simulink model "TRMS_MRAC_Node"  (R2024a)
settings: Solver=ode1  StartTime=0.0  StopTime=inf  FixedStep=0.01  RelTol=1e-3
model workspace (MAT data in the model file):
  alpha_gain = Simulink.Parameter
  alpha_gain.Value = 0.98
  alpha_gain.Complexity = 'real'
  alpha_gain.Dimensions = [1 1]
  alpha_gain.DataType = 'auto'
undefined symbols (not defined in the file or in its folder): A, B, C, D, DiscIntNeverNeededParam, P, pin_number, state, theta_theta
libraries: ros2lib x17, dspstat3 x1, sharedutil x1
settings Model: Creator=dsai9  LastModifiedBy=dsai9
settings OptimizationCC: EnhancedBackFolding=on  PassReuseOutputArgsAs=Individual arguments  ZeroExternalMemoryAtStartup=off  ZeroInternalMemoryAtStartup=off  MaxStackSize=64  OptimizeBlockOrder=speed  DifferentSizesBufferReuse=on  OptimizationCustomize=off  EfficientTunableParamExpr=on
settings DebuggingCC: ParameterTunabilityLossMsg=error
settings SFSimCC: MATLABDynamicMemAlloc=off
settings RTWCC: Description=Embedded Coder  SystemTargetFile=ert.tlc  HardwareBoard=Robot Operating System 2 (ROS 2)  TLCOptions="-aInlineSetEventsForThisBaseRateFcn=TLC_FALSE -aSuppressMultiTaskScheduler=TLC_FALSE  -aRateBasedStepFcn=0"  TemplateMakefile=ert_default_tmf  Toolchain=Colcon Tools  TargetLang=C++
settings CodeAppCC: ForceParamTrailComments=on  IgnoreCustomStorageClasses=off  OperatorAnnotations=on  SimulinkDataObjDesc=on  SFDataObjDesc=on  InsertBlockDesc=on
settings ERTTargetCC: CodeInterfacePackaging=C++ class  SupportContinuousTime=on  RootIOFormat=Structure reference

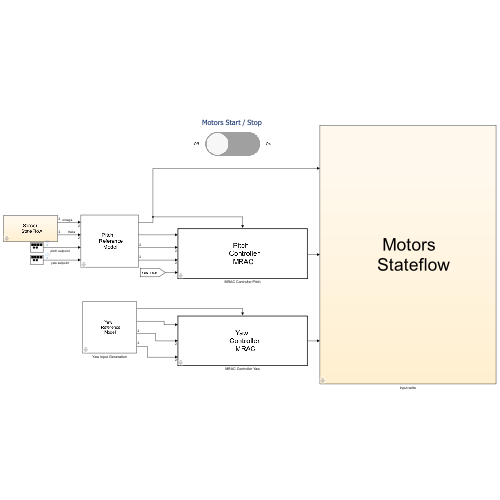
[thumbnail: Simulink's stored preview of the top-level diagram]
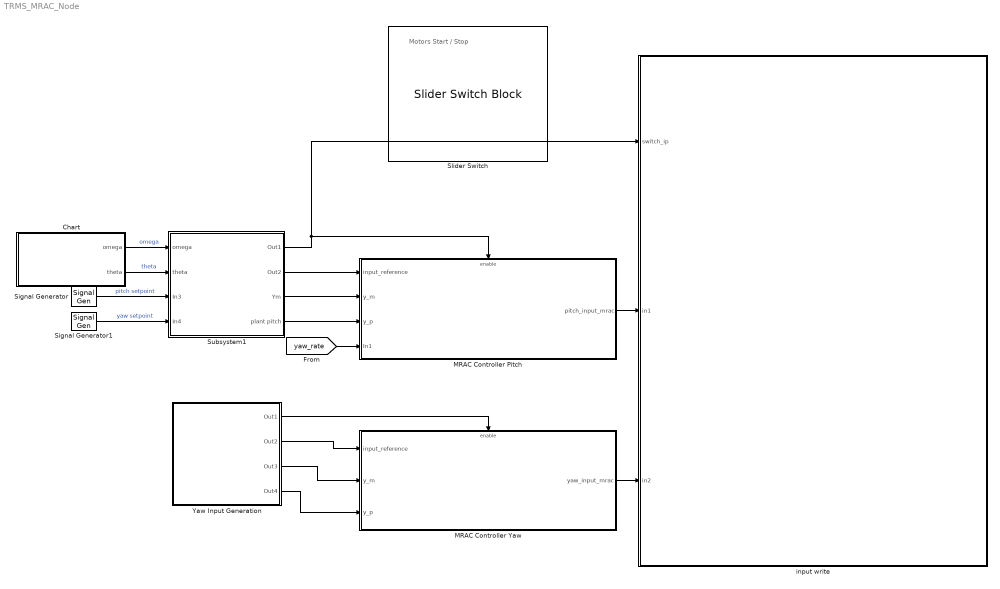
== system TRMS_MRAC_Node ==
  note: Motors Start / Stop
  Chart : Stateflow chart  TreatAsAtomicUnit=on
  MRAC Controller Pitch : Subsystem
  MRAC Controller Yaw : Subsystem
  Signal Generator : SignalGenerator  Amplitude=0  Frequency=0.5  Units=rad/sec
  Signal Generator1 : SignalGenerator  Amplitude=0  Frequency=0.5  Units=rad/sec
  Slider Switch : SliderSwitchBlock  LabelPosition=Hide
      settings: Values={{'Off', 'On'}, [0 1]}
  Subsystem1 : Subsystem
  Yaw Input Generation : Subsystem
  input write : Stateflow chart  TreatAsAtomicUnit=on
  wires:
  Yaw Input Generation/1(Out1) -> MRAC Controller Yaw/Enable
  Yaw Input Generation/2(Out2) -> MRAC Controller Yaw/1(input_reference)
  Yaw Input Generation/3(Out3) -> MRAC Controller Yaw/2(y_m)
  Yaw Input Generation/4(Out4) -> MRAC Controller Yaw/3(y_p)
  MRAC Controller Pitch/1(pitch_input_mrac) -> input write/2(in1)
  MRAC Controller Yaw/1(yaw_input_mrac) -> input write/3(in2)
  Chart/1(omega) -> Subsystem1/1(omega)  "omega"
  Chart/2(theta) -> Subsystem1/2(theta)  "theta"
  Signal Generator/1 -> Subsystem1/3(In3)  "pitch setpoint"
  Signal Generator1/1 -> Subsystem1/4(In4)  "yaw setpoint"
  Subsystem1/1(Out1) -> MRAC Controller Pitch/Enable, input write/1(switch_ip)
  Subsystem1/2(Out2) -> MRAC Controller Pitch/1(input_reference)
  Subsystem1/3(Ym) -> MRAC Controller Pitch/2(y_m)
  Subsystem1/4(plant pitch) -> MRAC Controller Pitch/3(y_p)
  [yaw_rate] -> MRAC Controller Pitch/4(In1)

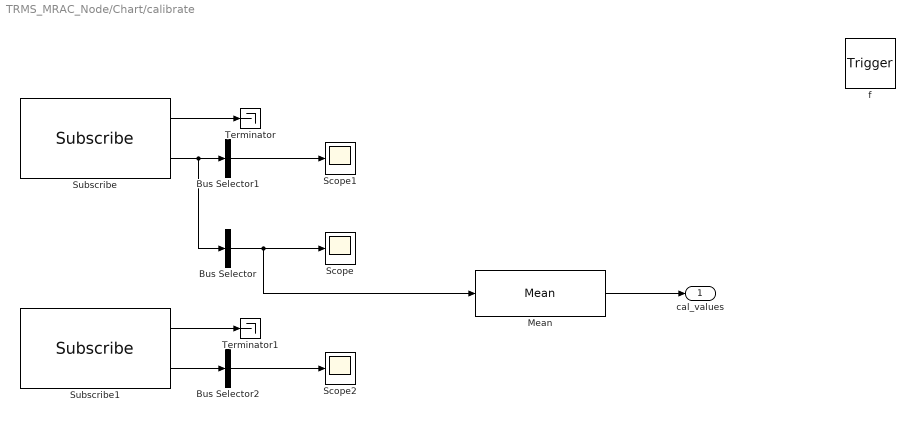
== system TRMS_MRAC_Node/Chart/calibrate ==
  f : TriggerPort  TriggerType=function-call  VariantControl=(inherit)
      settings: CopyFcn=Stateflow.SLINSF.SimulinkMan.removeBlockPreDeleteFcn  PreDeleteFcn=Stateflow.SLINSF.SimulinkMan.unsafePredeleteFcn
  Bus Selector : BusSelector  OutputSignals=angular_velocity.x,angular_velocity.y,angular_velocity.z  OutputAsBus=on
  Bus Selector1 : BusSelector  OutputSignals=linear_acceleration.x,linear_acceleration.y,linear_acceleration.z  OutputAsBus=on
  Bus Selector2 : BusSelector  OutputSignals=magnetic_field.x,magnetic_field.y,magnetic_field.z  OutputAsBus=on
  Mean : dspstat3/Mean  run=on  reset_popup=None  directionMode=Entire input  dimension=1  roiEnable=off  roiType=Rectangles  roiPortion=Entire ROI  roiOutput=Individual statistics for each ROI  roiFlag=off  roundingMode=Floor  overflowMode=off  outputDataTypeStr=Inherit: Same as accumulator  outputMin=[]  outputMax=[]  outputLastDataTypeStr=Inherit: Same as accumulator
  Scope : Scope
  Scope1 : Scope
  Scope2 : Scope
  Subscribe : ros2lib/Subscribe  topicSource=Select from ROS network  topic=/imu/data  messageType=sensor_msgs/Imu  sampleTime=-1  QOSHistory=Keep last  QOSDepth=1  QOSReliability=Reliable  QOSDurability=Volatile  QOSDeadline=Inf  QOSLifespan=Inf  QOSLiveliness=Automatic  QOSLeaseDuration=Inf  QOSAvoidROSNamespaceConventions=off
  Subscribe1 : ros2lib/Subscribe  topicSource=Select from ROS network  topic=/mag/data  messageType=sensor_msgs/MagneticField  sampleTime=-1  QOSHistory=Keep last  QOSDepth=1  QOSReliability=Reliable  QOSDurability=Volatile  QOSDeadline=Inf  QOSLifespan=Inf  QOSLiveliness=Automatic  QOSLeaseDuration=Inf  QOSAvoidROSNamespaceConventions=off
  Terminator : Terminator
  Terminator1 : Terminator
  cal_values : Outport  PortDimensions=3
  wires:
  Subscribe1/2 -> Bus Selector2/1
  Bus Selector2/1 -> Scope2/1
  Subscribe/1 -> Terminator/1
  Mean/1 -> cal_values/1
  Subscribe/2 -> Bus Selector/1, Bus Selector1/1
  Subscribe1/1 -> Terminator1/1
  Bus Selector/1 -> Mean/1, Scope/1
  Bus Selector1/1 -> Scope1/1

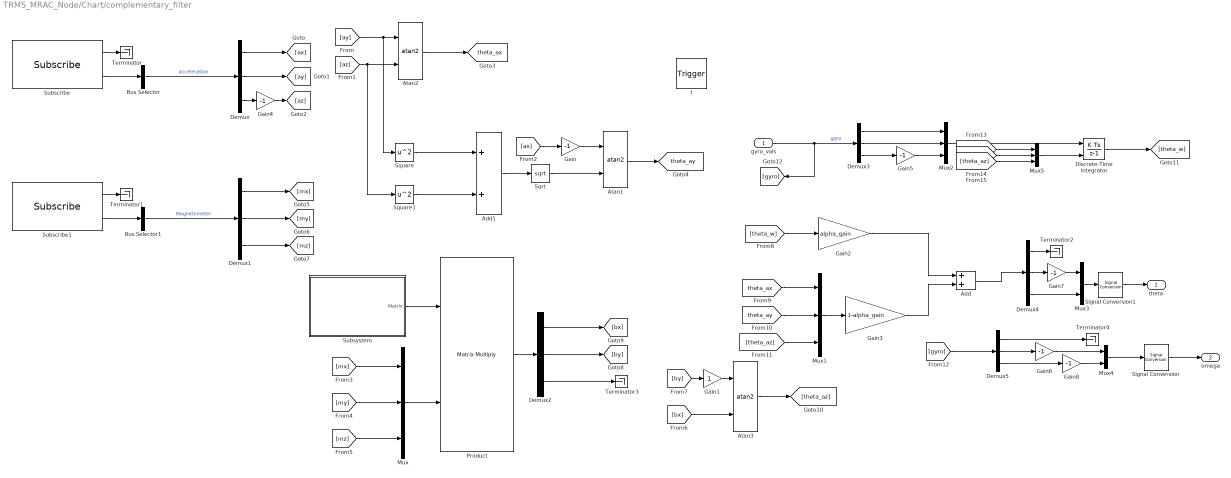
== system TRMS_MRAC_Node/Chart/complementary_filter ==
  gyro_vals : Inport  OutDataTypeStr=double  PortDimensions=3
  f : TriggerPort  TriggerType=function-call  VariantControl=(inherit)
      settings: CopyFcn=Stateflow.SLINSF.SimulinkMan.removeBlockPreDeleteFcn  PreDeleteFcn=Stateflow.SLINSF.SimulinkMan.unsafePredeleteFcn
  Add : Sum
  Add1 : Sum
  Atan1 : Trigonometry  Operator=atan2
  Atan2 : Trigonometry  Operator=atan2
  Atan3 : Trigonometry  Operator=atan2
  Bus Selector : BusSelector  OutputSignals=linear_acceleration.x,linear_acceleration.y,linear_acceleration.z  OutputAsBus=on
  Bus Selector1 : BusSelector  OutputSignals=magnetic_field.x,magnetic_field.y,magnetic_field.z  OutputAsBus=on
  Demux{,1..5} (6 alike) : Demux  Outputs=3
  Discrete-Time Integrator : DiscreteIntegrator  InitialConditionSource=external  SampleTime=-1  ICPrevOutput=DiscIntNeverNeededParam  ICPrevScaledInput=DiscIntNeverNeededParam
  Gain{,4..8} (6 alike) : Gain  Gain=-1
  Gain1 : Gain
  Gain2 : Gain  Gain=alpha_gain
  Gain3 : Gain  Gain=1-alpha_gain
  Mux{,1..2,5} (4 alike) : Mux  Inputs=3
  Mux3 : Mux  Inputs=2
  Mux4 : Mux  Inputs=2
  Product : Product  Multiplication=Matrix(*)
  Signal Conversion : SignalConversion  OverrideOpt=off
  Signal Conversion1 : SignalConversion  OverrideOpt=off
  Sqrt : Sqrt
  Square : Math  Operator=square
  Square1 : Math  Operator=square
  Subscribe : ros2lib/Subscribe  topicSource=Select from ROS network  topic=/imu/data  messageType=sensor_msgs/Imu  sampleTime=-1  QOSHistory=Keep last  QOSDepth=1  QOSReliability=Reliable  QOSDurability=Volatile  QOSDeadline=Inf  QOSLifespan=Inf  QOSLiveliness=Automatic  QOSLeaseDuration=Inf  QOSAvoidROSNamespaceConventions=off
  Subscribe1 : ros2lib/Subscribe  topicSource=Select from ROS network  topic=/mag/data  messageType=sensor_msgs/MagneticField  sampleTime=-1  QOSHistory=Keep last  QOSDepth=1  QOSReliability=Reliable  QOSDurability=Volatile  QOSDeadline=Inf  QOSLifespan=Inf  QOSLiveliness=Automatic  QOSLeaseDuration=Inf  QOSAvoidROSNamespaceConventions=off
  Subsystem : Subsystem
  Terminator{,1..4} (5 alike) : Terminator
  theta : Outport  PortDimensions=2
  omega : Outport  Port=2  PortDimensions=2
  tag scope: theta_ax=global, theta_ay=global
  wires:
  Subscribe/2 -> Bus Selector/1
  Subscribe1/2 -> Bus Selector1/1
  Bus Selector/1 -> Demux/1  "acceleration"
  Bus Selector1/1 -> Demux1/1  "Magnetometer"
  Subscribe/1 -> Terminator/1
  Subscribe1/1 -> Terminator1/1
  Demux/1 -> [ax]
  Demux/2 -> [ay]
  Demux/3 -> Gain4/1
  [ay] -> Square/1, Atan2/1
  [az] -> Square1/1, Atan2/2
  Atan2/1 -> [theta_ax]
  Square/1 -> Add1/1
  Square1/1 -> Add1/2
  Add1/1 -> Sqrt/1
  Sqrt/1 -> Atan1/2
  [ax] -> Gain/1
  Gain/1 -> Atan1/1
  Atan1/1 -> [theta_ay]
  Demux1/1 -> [mx]
  Demux1/2 -> [my]
  Demux1/3 -> [mz]
  Subsystem/1(Matrix) -> Product/1
  [mx] -> Mux/1
  [my] -> Mux/2
  [mz] -> Mux/3
  Mux/1 -> Product/2
  Product/1 -> Demux2/1
  Demux2/2 -> [by]
  Demux2/1 -> [bx]
  Demux2/3 -> Terminator3/1
  Gain1/1 -> Atan3/1
  [by] -> Gain1/1
  [bx] -> Atan3/2
  Atan3/1 -> [theta_az]
  Discrete-Time Integrator/1 -> [theta_w]
  [theta_w] -> Gain2/1
  [theta_ay] -> Mux1/2
  [theta_ax] -> Mux1/1
  [theta_az] -> Mux1/3
  Mux1/1 -> Gain3/1
  Gain2/1 -> Add/1
  Gain3/1 -> Add/2
  Gain4/1 -> [az]
  gyro_vals/1 -> Demux3/1, [gyro]  "gyro"
  Demux3/3 -> Gain5/1
  Gain5/1 -> Mux2/3
  Demux3/2 -> Mux2/2
  Demux3/1 -> Mux2/1
  Mux2/1 -> Discrete-Time Integrator/1
  Add/1 -> Demux4/1
  Mux3/1 -> Signal Conversion1/1
  Demux4/2 -> Gain7/1
  Demux4/3 -> Mux3/2
  Demux4/1 -> Terminator2/1
  Demux5/1 -> Terminator4/1
  Demux5/3 -> Gain8/1
  Demux5/2 -> Gain6/1
  [gyro] -> Demux5/1
  Mux4/1 -> Signal Conversion/1
  [theta_ax] -> Mux5/1
  [theta_ay] -> Mux5/2
  [theta_az] -> Mux5/3
  Mux5/1 -> Discrete-Time Integrator/2
  Gain6/1 -> Mux4/1
  Signal Conversion/1 -> omega/1
  Gain7/1 -> Mux3/1
  Gain8/1 -> Mux4/2
  Signal Conversion1/1 -> theta/1

== system TRMS_MRAC_Node/Chart/get_feedback ==
  cal_values : Inport  OutDataTypeStr=double  PortDimensions=3
  f : TriggerPort  TriggerType=function-call  VariantControl=(inherit)
      settings: CopyFcn=Stateflow.SLINSF.SimulinkMan.removeBlockPreDeleteFcn  PreDeleteFcn=Stateflow.SLINSF.SimulinkMan.unsafePredeleteFcn
  Add : Sum  Inputs=-+
  Bus Selector : BusSelector  OutputSignals=angular_velocity.x,angular_velocity.y,angular_velocity.z  OutputAsBus=on
  Subscribe : ros2lib/Subscribe  topicSource=Select from ROS network  topic=/imu/data  messageType=sensor_msgs/Imu  sampleTime=-1  QOSHistory=Keep last  QOSDepth=1  QOSReliability=Reliable  QOSDurability=Volatile  QOSDeadline=Inf  QOSLifespan=Inf  QOSLiveliness=Automatic  QOSLeaseDuration=Inf  QOSAvoidROSNamespaceConventions=off
  gyro_values : Outport
  wires:
  Subscribe/2 -> Bus Selector/1
  Bus Selector/1 -> Add/2
  cal_values/1 -> Add/1
  Add/1 -> gyro_values/1

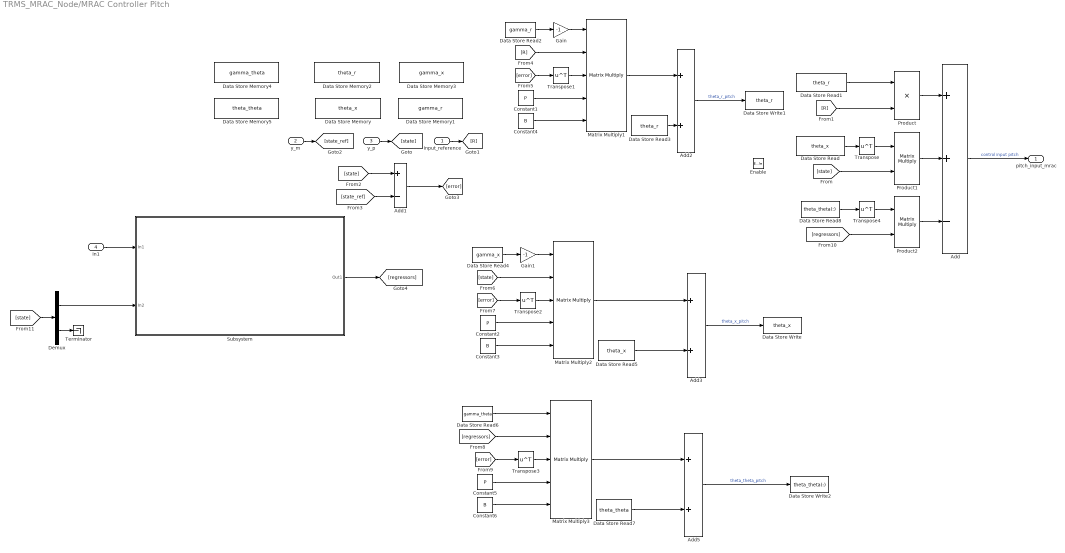
== system TRMS_MRAC_Node/MRAC Controller Pitch ==
  input_reference : Inport
  y_m : Inport  Port=2
  y_p : Inport  Port=3
  In1 : Inport  Port=4
  Enable : EnablePort
  Add : Sum  Inputs=++-
  Add1 : Sum  Inputs=+-
  Add2 : Sum
  Add3 : Sum
  Add5 : Sum
  Constant1 : Constant  Value=P
  Constant2 : Constant  Value=P
  Constant3 : Constant  Value=B
  Constant4 : Constant  Value=B
  Constant5 : Constant  Value=P
  Constant6 : Constant  Value=B
  Data Store Memory : DataStoreMemory  DataStoreName=theta_x  WriteAfterWriteMsg=warning  InitialValue=rand(1,2)  ShowAdditionalParam=off  Dimensions=[1,2]
  Data Store Memory1 : DataStoreMemory  DataStoreName=gamma_r  WriteAfterWriteMsg=warning  InitialValue=1  ShowAdditionalParam=off
  Data Store Memory2 : DataStoreMemory  DataStoreName=theta_r  WriteAfterWriteMsg=warning  InitialValue=rand(1,1)  ShowAdditionalParam=off  Dimensions=1
  Data Store Memory3 : DataStoreMemory  DataStoreName=gamma_x  WriteAfterWriteMsg=warning  InitialValue=ones(2,2)  ShowAdditionalParam=off
  Data Store Memory4 : DataStoreMemory  DataStoreName=gamma_theta  WriteAfterWriteMsg=warning  InitialValue=ones(2,2)  ShowAdditionalParam=off
  Data Store Memory5 : DataStoreMemory  DataStoreName=theta_theta  WriteAfterWriteMsg=warning  InitialValue=rand(1,2)  ShowAdditionalParam=off  Dimensions=[1,2]
  Data Store Read : DataStoreRead  DataStoreName=theta_x  IndexOptions=Index vector (dialog)  Indices=1  OutputSizes=1
  Data Store Read1 : DataStoreRead  DataStoreName=theta_r  IndexOptions=Index vector (dialog)  Indices=1  OutputSizes=1
  Data Store Read2 : DataStoreRead  DataStoreName=gamma_r  IndexOptions=Index vector (dialog)  Indices=1  OutputSizes=1
  Data Store Read3 : DataStoreRead  DataStoreName=theta_r  IndexOptions=Index vector (dialog)  Indices=1  OutputSizes=1
  Data Store Read4 : DataStoreRead  DataStoreName=gamma_x  IndexOptions=Index vector (dialog)  Indices=1  OutputSizes=1
  Data Store Read5 : DataStoreRead  DataStoreName=theta_x  IndexOptions=Index vector (dialog)  Indices=1  OutputSizes=1
  Data Store Read6 : DataStoreRead  DataStoreName=gamma_theta  IndexOptions=Index vector (dialog)  Indices=1  OutputSizes=1
  Data Store Read7 : DataStoreRead  DataStoreName=theta_theta  IndexOptions=Index vector (dialog)  Indices=1  OutputSizes=1
  Data Store Read8 : DataStoreRead  DataStoreName=theta_theta  DataStoreElements=theta_theta(:)  IndexOptions=Index vector (dialog)  Indices=1  OutputSizes=1
  Data Store Write : DataStoreWrite  DataStoreName=theta_x  DataStoreElements=theta_x  IndexOptions=Index vector (dialog)  Indices=1  OutputSizes=1
  Data Store Write1 : DataStoreWrite  DataStoreName=theta_r  DataStoreElements=theta_r  IndexOptions=Index vector (dialog)  Indices=1  OutputSizes=1
  Data Store Write2 : DataStoreWrite  DataStoreName=theta_theta  DataStoreElements=theta_theta(:)  IndexOptions=Index vector (dialog)  Indices=1  OutputSizes=1
  Demux : Demux  Outputs=2
  Gain : Gain  Gain=-1
  Gain1 : Gain  Gain=-1
  Matrix Multiply1 : Product  Inputs=5  Multiplication=Matrix(*)
  Matrix Multiply2 : Product  Inputs=5  Multiplication=Matrix(*)
  Matrix Multiply3 : Product  Inputs=5  Multiplication=Matrix(*)
  Product : Product
  Product1 : Product  Multiplication=Matrix(*)
  Product2 : Product  Multiplication=Matrix(*)
  Subsystem : Subsystem
  Terminator : Terminator
  Transpose{,1..4} (5 alike) : Math  Operator=transpose
  pitch_input_mrac : Outport
  wires:
  Product/1 -> Add/1
  Product1/1 -> Add/2
  Data Store Read1/1 -> Product/1
  y_p/1 -> [state]
  [state] -> Product1/2
  Data Store Read/1 -> Transpose/1
  input_reference/1 -> [R]
  y_m/1 -> [state_ref]
  [R] -> Product/2
  [state] -> Add1/1
  [state_ref] -> Add1/2
  Add1/1 -> [error]
  Data Store Read2/1 -> Gain/1
  Gain/1 -> Matrix Multiply1/1
  Data Store Read3/1 -> Add2/2
  Add2/1 -> Data Store Write1/1  "theta_r_pitch"
  Matrix Multiply1/1 -> Add2/1
  Transpose/1 -> Product1/1
  Matrix Multiply2/1 -> Add3/1
  Add3/1 -> Data Store Write/1  "theta_x_pitch"
  Data Store Read5/1 -> Add3/2
  Gain1/1 -> Matrix Multiply2/1
  Data Store Read4/1 -> Gain1/1
  [error] -> Transpose2/1
  Transpose2/1 -> Matrix Multiply2/3
  [state] -> Matrix Multiply2/2
  Constant2/1 -> Matrix Multiply2/4
  Constant3/1 -> Matrix Multiply2/5
  [R] -> Matrix Multiply1/2
  Transpose1/1 -> Matrix Multiply1/3
  [error] -> Transpose1/1
  Constant1/1 -> Matrix Multiply1/4
  Constant4/1 -> Matrix Multiply1/5
  Add/1 -> pitch_input_mrac/1  "control input pitch"
  Constant6/1 -> Matrix Multiply3/5
  Constant5/1 -> Matrix Multiply3/4
  [regressors] -> Matrix Multiply3/2
  Transpose3/1 -> Matrix Multiply3/3
  [error] -> Transpose3/1
  Data Store Read6/1 -> Matrix Multiply3/1
  Data Store Read7/1 -> Add5/2
  Add5/1 -> Data Store Write2/1  "theta_theta_pitch"
  Matrix Multiply3/1 -> Add5/1
  Subsystem/1(Out1) -> [regressors]
  Data Store Read8/1 -> Transpose4/1
  Transpose4/1 -> Product2/1
  Product2/1 -> Add/3
  [regressors] -> Product2/2
  In1/1 -> Subsystem/1(In1)
  Demux/1 -> Subsystem/2(In2)
  [state] -> Demux/1
  Demux/2 -> Terminator/1

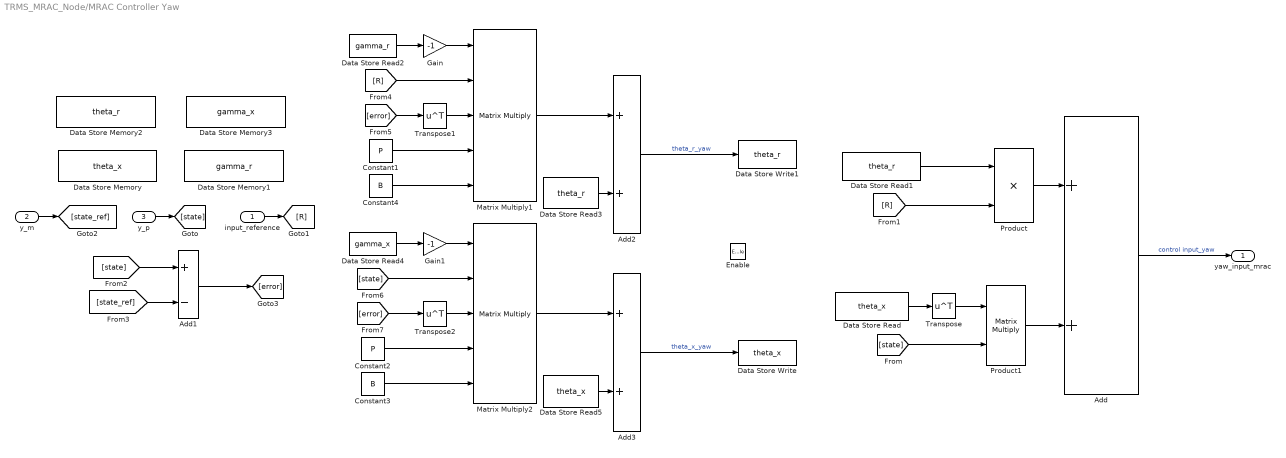
== system TRMS_MRAC_Node/MRAC Controller Yaw ==
  input_reference : Inport
  y_m : Inport  Port=2
  y_p : Inport  Port=3
  Enable : EnablePort
  Add : Sum
  Add1 : Sum  Inputs=+-
  Add2 : Sum
  Add3 : Sum
  Constant1 : Constant  Value=P
  Constant2 : Constant  Value=P
  Constant3 : Constant  Value=B
  Constant4 : Constant  Value=B
  Data Store Memory : DataStoreMemory  DataStoreName=theta_x  WriteAfterWriteMsg=warning  InitialValue=rand(1,2)  ShowAdditionalParam=off  Dimensions=[1,2]
  Data Store Memory1 : DataStoreMemory  DataStoreName=gamma_r  WriteAfterWriteMsg=warning  InitialValue=2  ShowAdditionalParam=off
  Data Store Memory2 : DataStoreMemory  DataStoreName=theta_r  WriteAfterWriteMsg=warning  InitialValue=rand(1,1)  ShowAdditionalParam=off  Dimensions=1
  Data Store Memory3 : DataStoreMemory  DataStoreName=gamma_x  WriteAfterWriteMsg=warning  InitialValue=3.*ones(2,2)  ShowAdditionalParam=off
  Data Store Read : DataStoreRead  DataStoreName=theta_x  IndexOptions=Index vector (dialog)  Indices=1  OutputSizes=1
  Data Store Read1 : DataStoreRead  DataStoreName=theta_r  IndexOptions=Index vector (dialog)  Indices=1  OutputSizes=1
  Data Store Read2 : DataStoreRead  DataStoreName=gamma_r  IndexOptions=Index vector (dialog)  Indices=1  OutputSizes=1
  Data Store Read3 : DataStoreRead  DataStoreName=theta_r  IndexOptions=Index vector (dialog)  Indices=1  OutputSizes=1
  Data Store Read4 : DataStoreRead  DataStoreName=gamma_x  IndexOptions=Index vector (dialog)  Indices=1  OutputSizes=1
  Data Store Read5 : DataStoreRead  DataStoreName=theta_x  IndexOptions=Index vector (dialog)  Indices=1  OutputSizes=1
  Data Store Write : DataStoreWrite  DataStoreName=theta_x  DataStoreElements=theta_x  IndexOptions=Index vector (dialog)  Indices=1  OutputSizes=1
  Data Store Write1 : DataStoreWrite  DataStoreName=theta_r  DataStoreElements=theta_r  IndexOptions=Index vector (dialog)  Indices=1  OutputSizes=1
  Gain : Gain  Gain=-1
  Gain1 : Gain  Gain=-1
  Matrix Multiply1 : Product  Inputs=5  Multiplication=Matrix(*)
  Matrix Multiply2 : Product  Inputs=5  Multiplication=Matrix(*)
  Product : Product
  Product1 : Product  Multiplication=Matrix(*)
  Transpose : Math  Operator=transpose
  Transpose1 : Math  Operator=transpose
  Transpose2 : Math  Operator=transpose
  yaw_input_mrac : Outport
  wires:
  Constant4/1 -> Matrix Multiply1/5
  Constant1/1 -> Matrix Multiply1/4
  [error] -> Transpose1/1
  Transpose1/1 -> Matrix Multiply1/3
  [R] -> Matrix Multiply1/2
  Constant3/1 -> Matrix Multiply2/5
  Constant2/1 -> Matrix Multiply2/4
  [state] -> Matrix Multiply2/2
  Transpose2/1 -> Matrix Multiply2/3
  [error] -> Transpose2/1
  Data Store Read4/1 -> Gain1/1
  Gain1/1 -> Matrix Multiply2/1
  Data Store Read5/1 -> Add3/2
  Add3/1 -> Data Store Write/1  "theta_x_yaw"
  Matrix Multiply2/1 -> Add3/1
  Add/1 -> yaw_input_mrac/1  "control input_yaw"
  Transpose/1 -> Product1/1
  Matrix Multiply1/1 -> Add2/1
  Add2/1 -> Data Store Write1/1  "theta_r_yaw"
  Data Store Read3/1 -> Add2/2
  Gain/1 -> Matrix Multiply1/1
  Data Store Read2/1 -> Gain/1
  Add1/1 -> [error]
  [state_ref] -> Add1/2
  [state] -> Add1/1
  [R] -> Product/2
  y_m/1 -> [state_ref]
  input_reference/1 -> [R]
  Data Store Read/1 -> Transpose/1
  [state] -> Product1/2
  y_p/1 -> [state]
  Data Store Read1/1 -> Product/1
  Product1/1 -> Add/2
  Product/1 -> Add/1

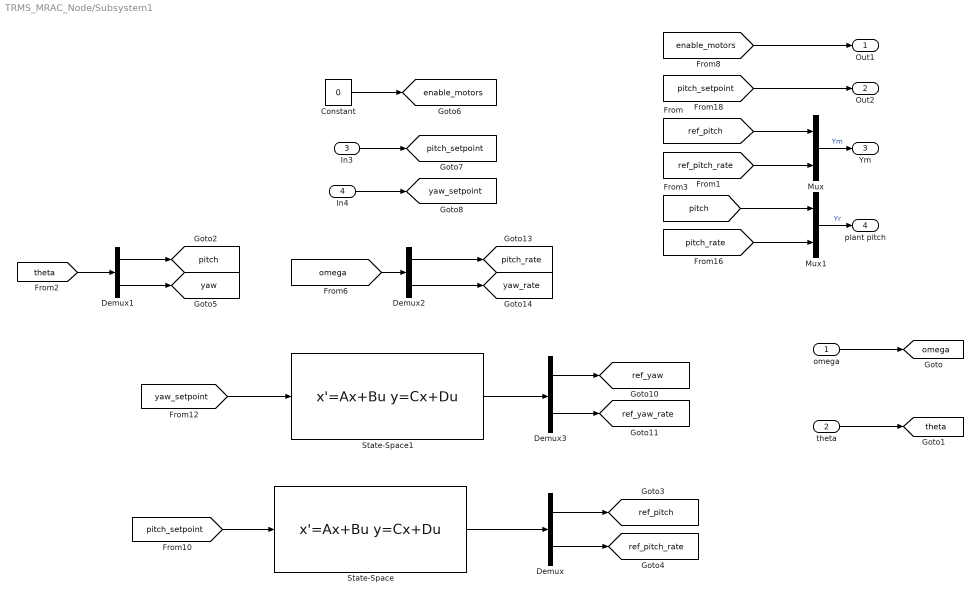
== system TRMS_MRAC_Node/Subsystem1 ==
  omega : Inport
  theta : Inport  Port=2
  In3 : Inport  Port=3
  In4 : Inport  Port=4
  Constant : Constant  Value=0
  Demux{,1..3} (4 alike) : Demux  Outputs=2
  Mux : Mux  Inputs=2
  Mux1 : Mux  Inputs=2
  State-Space : StateSpace  A=A  B=B  C=C  D=D  InitialCondition=[-0.6; 0]
  State-Space1 : StateSpace  A=A  B=B  C=C  D=D  InitialCondition=[-0.6; 0]
  Out1 : Outport
  Out2 : Outport  Port=2
  Ym : Outport  Port=3
  plant pitch : Outport  Port=4
  tag scope: enable_motors=global, omega=global, pitch=global, pitch_rate=global, pitch_setpoint=global, ref_pitch=global, ref_pitch_rate=global, ref_yaw=global, ref_yaw_rate=global, theta=global, yaw=global, yaw_rate=global, yaw_setpoint=global
  wires:
  Demux/1 -> [ref_pitch]
  [ref_pitch] -> Mux/1
  Demux3/2 -> [ref_yaw_rate]
  State-Space1/1 -> Demux3/1
  Demux3/1 -> [ref_yaw]
  [ref_pitch_rate] -> Mux/2
  [pitch] -> Mux1/1
  [pitch_setpoint] -> Out2/1
  [pitch_setpoint] -> State-Space/1
  [omega] -> Demux2/1
  Demux2/2 -> [yaw_rate]
  [pitch_rate] -> Mux1/2
  Demux2/1 -> [pitch_rate]
  Demux/2 -> [ref_pitch_rate]
  State-Space/1 -> Demux/1
  Constant/1 -> [enable_motors]
  [enable_motors] -> Out1/1
  Mux1/1 -> plant pitch/1  "Yr"
  Mux/1 -> Ym/1  "Ym"
  omega/1 -> [omega]
  theta/1 -> [theta]
  In4/1 -> [yaw_setpoint]
  In3/1 -> [pitch_setpoint]
  [yaw_setpoint] -> State-Space1/1
  [theta] -> Demux1/1
  Demux1/1 -> [pitch]
  Demux1/2 -> [yaw]

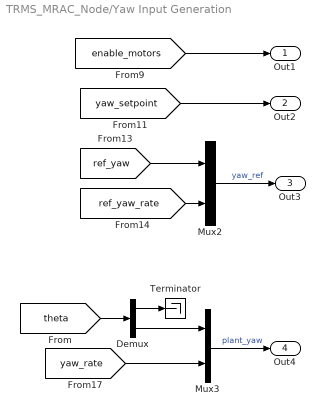
== system TRMS_MRAC_Node/Yaw Input Generation ==
  Demux : Demux  Outputs=2
  Mux2 : Mux  Inputs=2
  Mux3 : Mux  Inputs=2
  Terminator : Terminator
  Out1 : Outport
  Out2 : Outport  Port=2
  Out3 : Outport  Port=3
  Out4 : Outport  Port=4
  wires:
  [ref_yaw] -> Mux2/1
  [enable_motors] -> Out1/1
  Mux2/1 -> Out3/1  "yaw_ref"
  [ref_yaw_rate] -> Mux2/2
  Mux3/1 -> Out4/1  "plant_yaw"
  [yaw_setpoint] -> Out2/1
  Demux/2 -> Mux3/1
  [yaw_rate] -> Mux3/2
  [theta] -> Demux/1
  Demux/1 -> Terminator/1

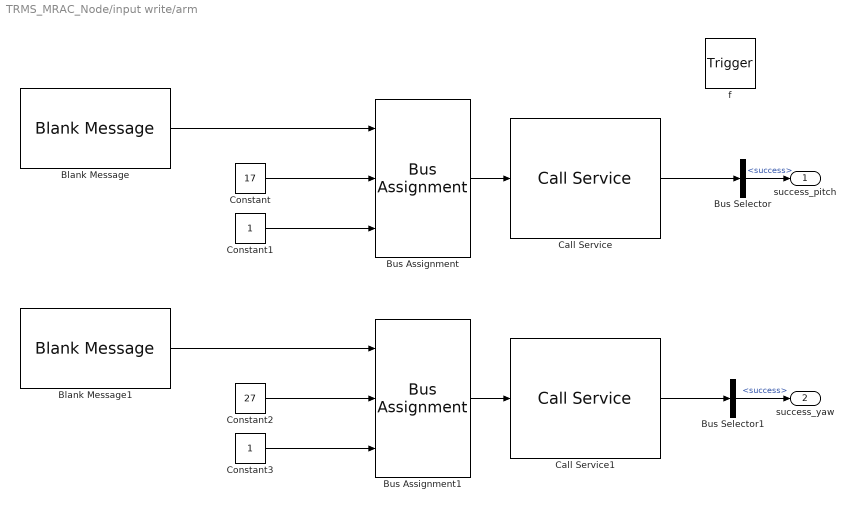
== system TRMS_MRAC_Node/input write/arm ==
  f : TriggerPort  TriggerType=function-call  VariantControl=(inherit)
      settings: CopyFcn=Stateflow.SLINSF.SimulinkMan.removeBlockPreDeleteFcn  PreDeleteFcn=Stateflow.SLINSF.SimulinkMan.unsafePredeleteFcn
  Blank Message : ros2lib/Blank Message  messageClass=Service Request  entityType=aerobot_interfaces/EscSrv  messageType=aerobot_interfaces/EscSrvRequest  SampleTime=inf
  Blank Message1 : ros2lib/Blank Message  messageClass=Service Request  entityType=aerobot_interfaces/EscSrv  messageType=aerobot_interfaces/EscSrvRequest  SampleTime=inf
  Bus Assignment : BusAssignment  AssignedSignals=pin_number,state
  Bus Assignment1 : BusAssignment  AssignedSignals=pin_number,state
  Bus Selector : BusSelector  OutputSignals=success
  Bus Selector1 : BusSelector  OutputSignals=success
  Call Service : ros2lib/Call Service  topicSource=Select from ROS network  service=/arm_pitch  serviceType=aerobot_interfaces/EscSrv  connectionTimeout=5  ShowErrorCodeOutput=off  legacyBusStruct=off  QOSHistory=Keep last  QOSDepth=1  QOSReliability=Reliable  QOSDurability=Volatile  QOSDeadline=Inf  QOSLifespan=Inf  QOSLiveliness=Automatic  QOSLeaseDuration=Inf  QOSAvoidROSNamespaceConventions=off
  Call Service1 : ros2lib/Call Service  topicSource=Select from ROS network  service=/arm_pitch  serviceType=aerobot_interfaces/EscSrv  connectionTimeout=5  ShowErrorCodeOutput=off  legacyBusStruct=off  QOSHistory=Keep last  QOSDepth=1  QOSReliability=Reliable  QOSDurability=Volatile  QOSDeadline=Inf  QOSLifespan=Inf  QOSLiveliness=Automatic  QOSLeaseDuration=Inf  QOSAvoidROSNamespaceConventions=off
  Constant : Constant  Value=17  OutDataTypeStr=int8
  Constant1 : Constant  OutDataTypeStr=boolean
  Constant2 : Constant  Value=27  OutDataTypeStr=int8
  Constant3 : Constant  OutDataTypeStr=boolean
  success_pitch : Outport
  success_yaw : Outport  Port=2
  wires:
  Blank Message/1 -> Bus Assignment/1
  Bus Assignment/1 -> Call Service/1
  Constant/1 -> Bus Assignment/2
  Constant1/1 -> Bus Assignment/3
  Constant3/1 -> Bus Assignment1/3
  Blank Message1/1 -> Bus Assignment1/1
  Bus Assignment1/1 -> Call Service1/1
  Constant2/1 -> Bus Assignment1/2
  Call Service/1 -> Bus Selector/1
  Bus Selector/1 -> success_pitch/1  "<success>"
  Call Service1/1 -> Bus Selector1/1
  Bus Selector1/1 -> success_yaw/1  "<success>"

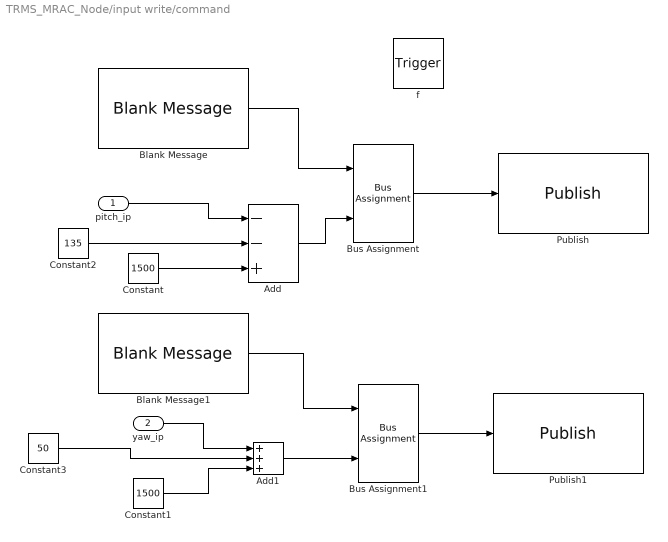
== system TRMS_MRAC_Node/input write/command ==
  pitch_ip : Inport  OutDataTypeStr=double  PortDimensions=1
  yaw_ip : Inport  Port=2  OutDataTypeStr=double  PortDimensions=1
  f : TriggerPort  TriggerType=function-call  VariantControl=(inherit)
      settings: CopyFcn=Stateflow.SLINSF.SimulinkMan.removeBlockPreDeleteFcn  PreDeleteFcn=Stateflow.SLINSF.SimulinkMan.unsafePredeleteFcn
  Add : Sum  Inputs=--+
  Add1 : Sum  Inputs=+++
  Blank Message : ros2lib/Blank Message  messageClass=Message  entityType=std_msgs/Float64  messageType=std_msgs/Float64  SampleTime=inf
  Blank Message1 : ros2lib/Blank Message  messageClass=Message  entityType=std_msgs/Float64  messageType=std_msgs/Float64  SampleTime=inf
  Bus Assignment : BusAssignment  AssignedSignals=data
  Bus Assignment1 : BusAssignment  AssignedSignals=data
  Constant : Constant  Value=1500
  Constant1 : Constant  Value=1500
  Constant2 : Constant  Value=135
  Constant3 : Constant  Value=50
  Publish : ros2lib/Publish  topicSource=Select from ROS network  topic=/esc_command1  messageType=std_msgs/Float64  QOSHistory=Keep last  QOSDepth=1  QOSReliability=Reliable  QOSDurability=Volatile  QOSDeadline=Inf  QOSLifespan=Inf  QOSLiveliness=Automatic  QOSLeaseDuration=Inf  QOSAvoidROSNamespaceConventions=off
  Publish1 : ros2lib/Publish  topicSource=Select from ROS network  topic=/esc_command2  messageType=std_msgs/Float64  QOSHistory=Keep last  QOSDepth=1  QOSReliability=Reliable  QOSDurability=Volatile  QOSDeadline=Inf  QOSLifespan=Inf  QOSLiveliness=Automatic  QOSLeaseDuration=Inf  QOSAvoidROSNamespaceConventions=off
  wires:
  Bus Assignment/1 -> Publish/1
  Blank Message/1 -> Bus Assignment/1
  Add/1 -> Bus Assignment/2
  Constant/1 -> Add/3
  yaw_ip/1 -> Add1/1
  Constant1/1 -> Add1/3
  Add1/1 -> Bus Assignment1/2
  Blank Message1/1 -> Bus Assignment1/1
  Bus Assignment1/1 -> Publish1/1
  Constant2/1 -> Add/2
  Constant3/1 -> Add1/2
  pitch_ip/1 -> Add/1

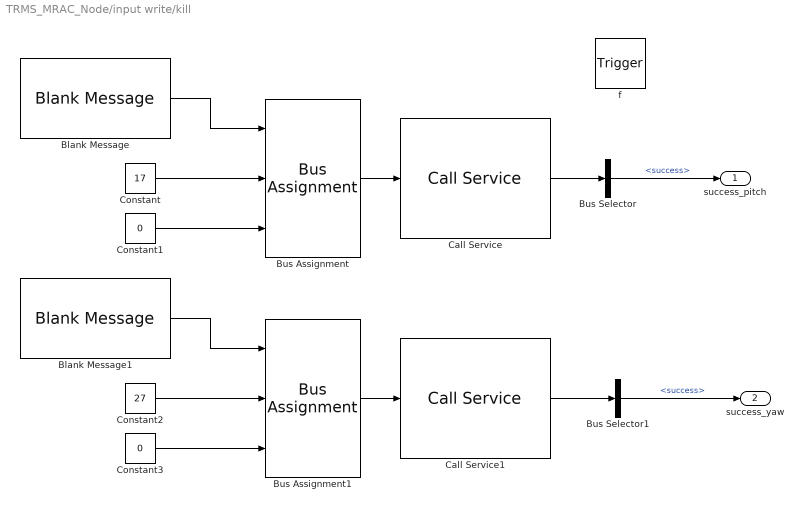
== system TRMS_MRAC_Node/input write/kill ==
  f : TriggerPort  TriggerType=function-call  VariantControl=(inherit)
      settings: CopyFcn=Stateflow.SLINSF.SimulinkMan.removeBlockPreDeleteFcn  PreDeleteFcn=Stateflow.SLINSF.SimulinkMan.unsafePredeleteFcn
  Blank Message : ros2lib/Blank Message  messageClass=Service Request  entityType=aerobot_interfaces/EscSrv  messageType=aerobot_interfaces/EscSrvRequest  SampleTime=inf
  Blank Message1 : ros2lib/Blank Message  messageClass=Service Request  entityType=aerobot_interfaces/EscSrv  messageType=aerobot_interfaces/EscSrvRequest  SampleTime=inf
  Bus Assignment : BusAssignment  AssignedSignals=pin_number,state
  Bus Assignment1 : BusAssignment  AssignedSignals=pin_number,state
  Bus Selector : BusSelector  OutputSignals=success
  Bus Selector1 : BusSelector  OutputSignals=success
  Call Service : ros2lib/Call Service  topicSource=Select from ROS network  service=/arm_pitch  serviceType=aerobot_interfaces/EscSrv  connectionTimeout=5  ShowErrorCodeOutput=off  legacyBusStruct=off  QOSHistory=Keep last  QOSDepth=1  QOSReliability=Reliable  QOSDurability=Volatile  QOSDeadline=Inf  QOSLifespan=Inf  QOSLiveliness=Automatic  QOSLeaseDuration=Inf  QOSAvoidROSNamespaceConventions=off
  Call Service1 : ros2lib/Call Service  topicSource=Select from ROS network  service=/arm_pitch  serviceType=aerobot_interfaces/EscSrv  connectionTimeout=5  ShowErrorCodeOutput=off  legacyBusStruct=off  QOSHistory=Keep last  QOSDepth=1  QOSReliability=Reliable  QOSDurability=Volatile  QOSDeadline=Inf  QOSLifespan=Inf  QOSLiveliness=Automatic  QOSLeaseDuration=Inf  QOSAvoidROSNamespaceConventions=off
  Constant : Constant  Value=17  OutDataTypeStr=int8
  Constant1 : Constant  Value=0  OutDataTypeStr=boolean
  Constant2 : Constant  Value=27  OutDataTypeStr=int8
  Constant3 : Constant  Value=0  OutDataTypeStr=boolean
  success_pitch : Outport
  success_yaw : Outport  Port=2
  wires:
  Blank Message/1 -> Bus Assignment/1
  Bus Assignment/1 -> Call Service/1
  Constant/1 -> Bus Assignment/2
  Constant1/1 -> Bus Assignment/3
  Call Service1/1 -> Bus Selector1/1
  Constant3/1 -> Bus Assignment1/3
  Blank Message1/1 -> Bus Assignment1/1
  Bus Assignment1/1 -> Call Service1/1
  Constant2/1 -> Bus Assignment1/2
  Call Service/1 -> Bus Selector/1
  Bus Selector/1 -> success_pitch/1  "<success>"
  Bus Selector1/1 -> success_yaw/1  "<success>"

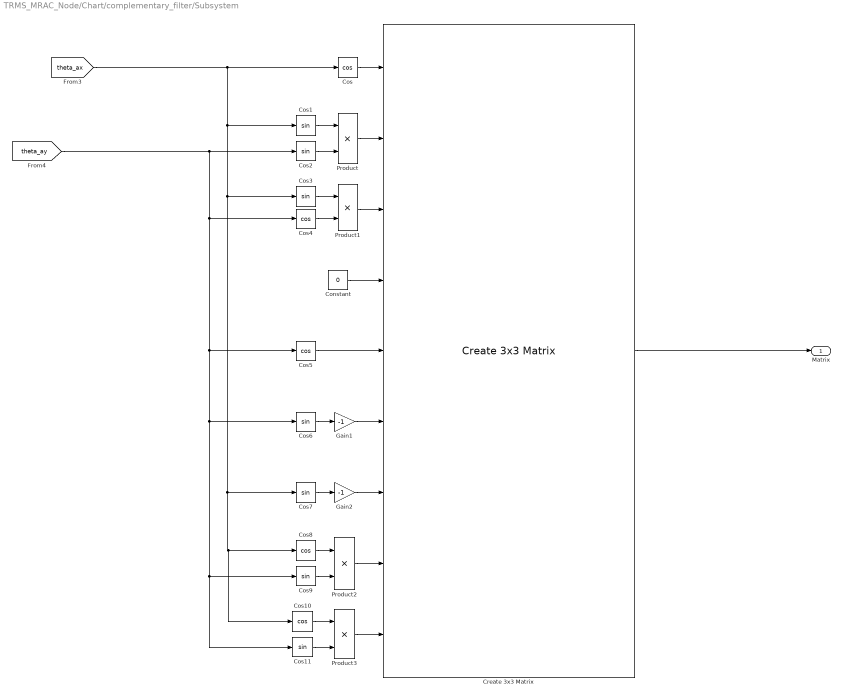
== system TRMS_MRAC_Node/Chart/complementary_filter/Subsystem ==
  Constant : Constant  Value=0
  Cos{,4..5,8,10} (5 alike) : Trigonometry  Operator=cos
  Cos{1..3,6..7,9,11} (7 alike) : Trigonometry
  Create 3x3 Matrix : sharedutil/Create 3x3 Matrix  aMode=aMode
      settings: LibrarySourceBlock=aerolibutil/Create 3x3 Matrix
  Gain1 : Gain  Gain=-1
  Gain2 : Gain  Gain=-1
  Product{,1..3} (4 alike) : Product
  Matrix : Outport  PortDimensions=[3,3]
  wires:
  Gain2/1 -> Create 3x3 Matrix/7
  Cos7/1 -> Gain2/1
  Cos8/1 -> Product2/1
  [theta_ax] -> Cos/1, Cos10/1, Cos8/1, Cos7/1, Cos3/1, Cos1/1
  Product3/1 -> Create 3x3 Matrix/9
  Cos11/1 -> Product3/2
  Cos9/1 -> Product2/2
  Cos10/1 -> Product3/1
  Constant/1 -> Create 3x3 Matrix/4
  Product/1 -> Create 3x3 Matrix/2
  Cos3/1 -> Product1/1
  [theta_ay] -> Cos5/1, Cos6/1, Cos11/1, Cos9/1, Cos4/1, Cos2/1
  Cos1/1 -> Product/1
  Cos6/1 -> Gain1/1
  Cos/1 -> Create 3x3 Matrix/1
  Product1/1 -> Create 3x3 Matrix/3
  Gain1/1 -> Create 3x3 Matrix/6
  Cos5/1 -> Create 3x3 Matrix/5
  Cos4/1 -> Product1/2
  Product2/1 -> Create 3x3 Matrix/8
  Cos2/1 -> Product/2
  Create 3x3 Matrix/1 -> Matrix/1

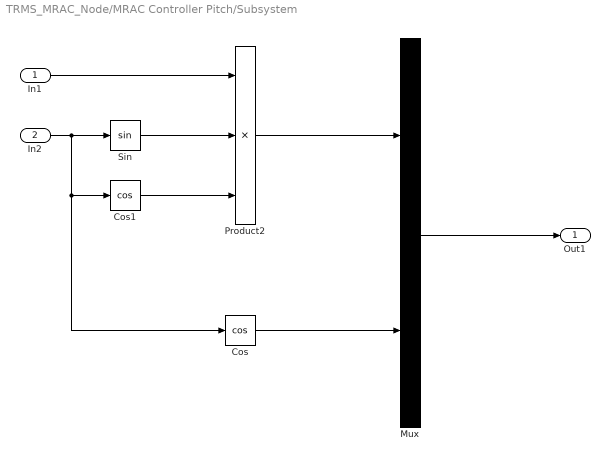
== system TRMS_MRAC_Node/MRAC Controller Pitch/Subsystem ==
  In1 : Inport
  In2 : Inport  Port=2
  Cos : Trigonometry  Operator=cos
  Cos1 : Trigonometry  Operator=cos
  Mux : Mux  Inputs=2
  Product2 : Product  Inputs=3
  Sin : Trigonometry
  Out1 : Outport
  wires:
  In2/1 -> Cos1/1, Cos/1, Sin/1
  Sin/1 -> Product2/2
  In1/1 -> Product2/1
  Cos1/1 -> Product2/3
  Product2/1 -> Mux/1
  Cos/1 -> Mux/2
  Mux/1 -> Out1/1

== stateflow chart TRMS_MRAC_Node/input write ==
  state [success_pitch,success_yaw] = kill [function]
  state command(pitch_ip,yaw_ip) [function]
  state [success_pitch,success_yaw] = arm [function]
  state arm_state
    entry:
    [ps, ys] = arm()
    move = 1
  state Command_state
    during:
    command(in1, in2)
  state kill_state
    entry:
    [ps, ys] = kill()
  (default) -> arm_state
  arm_state -> Command_state : [move == 1]
  Command_state -> kill_state : [switch_ip ==  0]
  kill_state -> arm_state : [switch_ip == 1]
  data: success_pitch function_output; success_yaw function_output; pitch_ip function_input double size=1; yaw_ip function_input double size=1; success_pitch function_output; success_yaw function_output; switch_ip input; in1 input; in2 input; ys local; ps local; move local

== stateflow chart TRMS_MRAC_Node/Chart ==
  state orientation_calculation
    during:
    gyro_values = get_feedback(cal_values);
    [theta, omega] = complementary_filter(gyro_values);
  state calibrate_start
    entry:
    calibrated = 0;
    i = 0;
    during:
    cal_values = calibrate();
    i = i + 1;
    if i == 100;
    disp('Calibration Done')
    calibrated = 1;
    end
  state cal_values = calibrate [function]
  state gyro_values = get_feedback(cal_values) [function]
  state [theta,omega] = complementary_filter(gyro_vals) [function]
  (default) -> calibrate_start
  calibrate_start -> orientation_calculation : [calibrated==1]
  data: cal_values function_output size=3; cal_values function_input double size=3; gyro_values function_output; gyro_vals function_input double size=3; theta function_output size=2; omega function_output size=2; calibrated local; i local; cal_values local; omega output; gyro_values local; theta output
